simulink library "Source_Lib"  (R2017a)
settings: Solver=VariableStepAuto  StartTime=0.0  StopTime=10.0  RelTol=1e-3
undefined symbols (not defined in the file or in its folder): Cmu0, delta0, fb, GOV1_K2, ia0, ib0, Ib2, ic0, pha0, phb0, phc0, Theta0_deg, Time_Step, V0_pu, Vfu0
libraries: powerlib x41, Control_Lib x14, spsPower3phInstantaneousLib x3, spsSynchronousMachinepuFundamentalLib x2
(part 2 of 2)

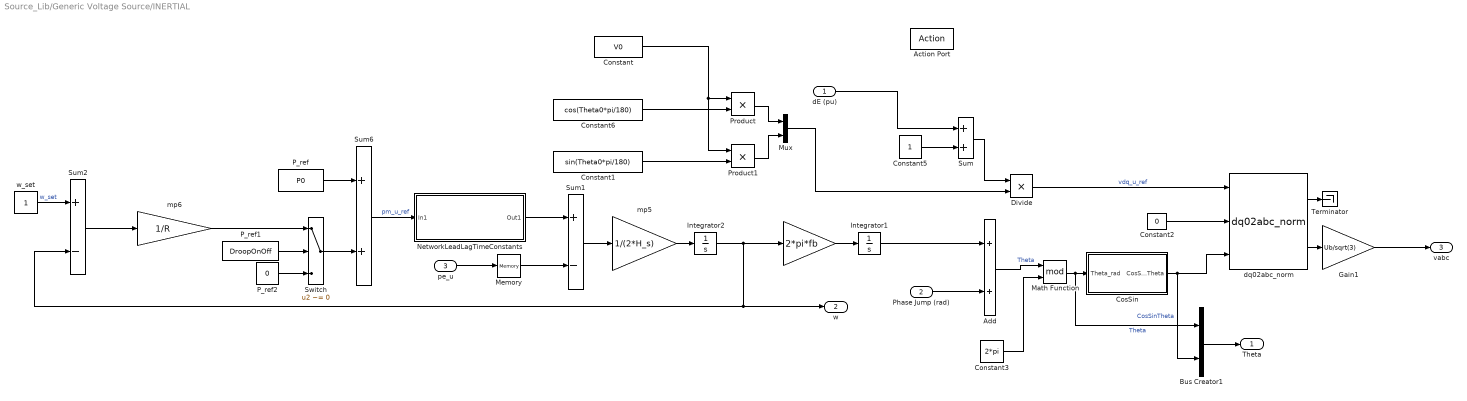
== system Source_Lib/Generic Voltage Source/INERTIAL ==
  dE (pu) : Inport
  Phase Jump (rad) : Inport  Port=2
  pe_u : Inport  Port=3
  Action Port : ActionPort
  " " : Gain  Gain=2*pi*fb
  Add : Sum
  Bus Creator1 : BusCreator  Inputs=2
  Constant : Constant  Value=V0
  Constant1 : Constant  Value=sin(Theta0*pi/180)
  Constant2 : Constant  Value=0
  Constant3 : Constant  Value=2*pi
  Constant5 : Constant
  Constant6 : Constant  Value=cos(Theta0*pi/180)
  CosSin : Subsystem
  Divide : Product  Inputs=**
  Gain1 : Gain  Gain=Ub/sqrt(3)
  Integrator1 : Integrator  InitialCondition=Theta0*pi/180
  Integrator2 : Integrator  InitialCondition=1
  Math Function : Math  Operator=mod  SaturateOnIntegerOverflow=on
  Memory : Memory
  Mux : Mux  Inputs=2
  NetworkLeadLagTimeConstants : Subsystem
  P_ref : Constant  Value=P0
  P_ref1 : Constant  Value=DroopOnOff
  P_ref2 : Constant  Value=0
  Product : Product
  Product1 : Product
  Sum : Sum
  Sum1 : Sum  Inputs=+-
  Sum2 : Sum  Inputs=+-
  Sum6 : Sum
  Switch : Switch  Criteria=u2 ~= 0
  Terminator : Terminator
  dq02abc_norm : Control_Lib/dq02abc_norm  referenceAxisMode=Reference axis at 90 degrees behind phase_a  baseUpdateGain=sqrt(3)
      settings: SourceProductName=VSC_Lib
  mp5 : Gain  Gain=1/(2*H_s)
  mp6 : Gain  Gain=1/R
  w_set : Constant
  Theta : Outport
  w : Outport  Port=2
  vabc : Outport  Port=3
  wires:
  dq02abc_norm/2 -> Gain1/1
  dE (pu)/1 -> Sum/1
  dq02abc_norm/1 -> Terminator/1
  Sum/1 -> Divide/1
  Gain1/1 -> vabc/1
  Product/1 -> Mux/1
  Constant6/1 -> Product/2
  Constant3/1 -> Math Function/2
  CosSin/1(CosSinTheta) -> Bus Creator1/2, dq02abc_norm/3  "CosSinTheta"
  Constant1/1 -> Product1/2
  Divide/1 -> dq02abc_norm/1  "vdq_u_ref"
  Constant/1 -> Product/1, Product1/1
  Phase Jump (rad)/1 -> Add/2
  Add/1 -> Math Function/1  "Theta"
  Math Function/1 -> Bus Creator1/1, CosSin/1(Theta_rad)  "Theta"
  Constant2/1 -> dq02abc_norm/2
  Product1/1 -> Mux/2
  Constant5/1 -> Sum/2
  Mux/1 -> Divide/2
  Bus Creator1/1 -> Theta/1
  NetworkLeadLagTimeConstants/1(Out1) -> Sum1/1
  P_ref/1 -> Sum6/1
  mp6/1 -> Switch/1
  " "/1 -> Integrator1/1
  Sum2/1 -> mp6/1
  P_ref2/1 -> Switch/3
  Integrator2/1 -> " "/1, Sum2/2, w/1
  P_ref1/1 -> Switch/2
  mp5/1 -> Integrator2/1
  pe_u/1 -> Memory/1
  Sum1/1 -> mp5/1
  Sum6/1 -> NetworkLeadLagTimeConstants/1(In1)  "pm_u_ref"
  Integrator1/1 -> Add/1
  Switch/1 -> Sum6/2
  w_set/1 -> Sum2/1  "w_set"
  Memory/1 -> Sum1/2

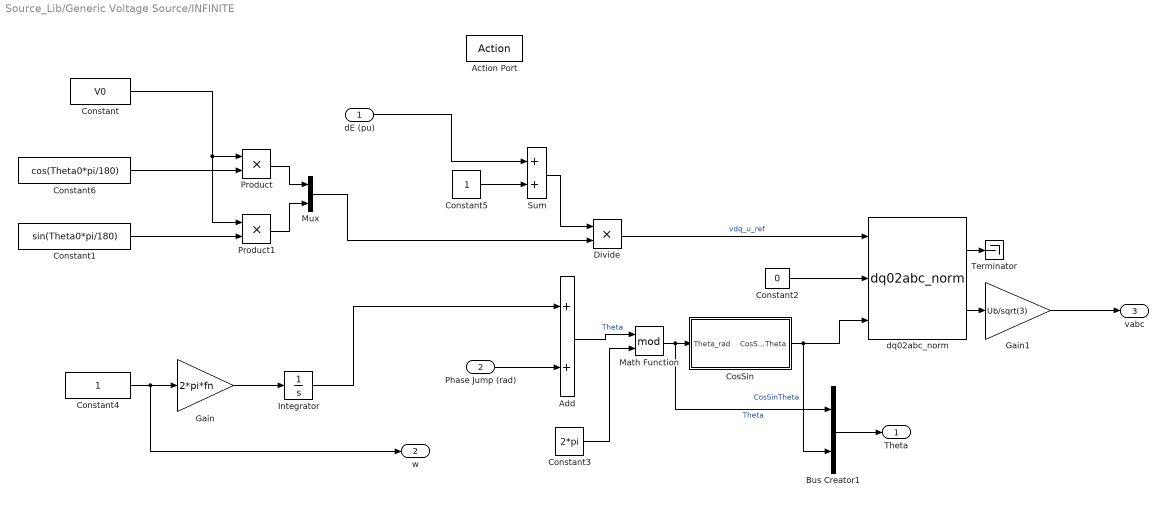
== system Source_Lib/Generic Voltage Source/INFINITE ==
  dE (pu) : Inport
  Phase Jump (rad) : Inport  Port=2
  Action Port : ActionPort
  Add : Sum
  Bus Creator1 : BusCreator  Inputs=2
  Constant : Constant  Value=V0
  Constant1 : Constant  Value=sin(Theta0*pi/180)
  Constant2 : Constant  Value=0
  Constant3 : Constant  Value=2*pi
  Constant4 : Constant
  Constant5 : Constant
  Constant6 : Constant  Value=cos(Theta0*pi/180)
  CosSin : Subsystem
  Divide : Product  Inputs=**
  Gain : Gain  Gain=2*pi*fn
  Gain1 : Gain  Gain=Ub/sqrt(3)
  Integrator : Integrator  InitialCondition=Theta0*pi/180
  Math Function : Math  Operator=mod  SaturateOnIntegerOverflow=on
  Mux : Mux  Inputs=2
  Product : Product
  Product1 : Product
  Sum : Sum
  Terminator : Terminator
  dq02abc_norm : Control_Lib/dq02abc_norm  referenceAxisMode=Reference axis at 90 degrees behind phase_a  baseUpdateGain=sqrt(3)
      settings: SourceProductName=VSC_Lib
  Theta : Outport
  w : Outport  Port=2
  vabc : Outport  Port=3
  wires:
  dq02abc_norm/2 -> Gain1/1
  Integrator/1 -> Add/1
  Gain/1 -> Integrator/1
  dE (pu)/1 -> Sum/1
  dq02abc_norm/1 -> Terminator/1
  Sum/1 -> Divide/1
  Constant4/1 -> w/1, Gain/1
  Gain1/1 -> vabc/1
  Product/1 -> Mux/1
  Constant6/1 -> Product/2
  Constant3/1 -> Math Function/2
  CosSin/1(CosSinTheta) -> Bus Creator1/2, dq02abc_norm/3  "CosSinTheta"
  Constant1/1 -> Product1/2
  Divide/1 -> dq02abc_norm/1  "vdq_u_ref"
  Constant/1 -> Product/1, Product1/1
  Phase Jump (rad)/1 -> Add/2
  Add/1 -> Math Function/1  "Theta"
  Math Function/1 -> Bus Creator1/1, CosSin/1(Theta_rad)  "Theta"
  Constant2/1 -> dq02abc_norm/2
  Product1/1 -> Mux/2
  Constant5/1 -> Sum/2
  Mux/1 -> Divide/2
  Bus Creator1/1 -> Theta/1

== system Source_Lib/Generic Voltage Source/Source_For_OP ==
  v_abc_ref : Inport
  Controlled Voltage Source1 : powerlib/Electrical Sources/Controlled Voltage Source  Initialize=off  Source_Type=AC  Amplitude=V0*Ub*sqrt(2/3)*sin(Theta0)  Phase=(Theta0*180/pi)  Frequency=fb  Measurements=None
  Controlled Voltage Source2 : powerlib/Electrical Sources/Controlled Voltage Source  Initialize=off  Source_Type=AC  Amplitude=V0*Ub*sqrt(2/3)*sin(Theta0-2*pi/3)  Phase=(Theta0*180/pi)-120  Frequency=fb  Measurements=None
  Controlled Voltage Source3 : powerlib/Electrical Sources/Controlled Voltage Source  Initialize=off  Source_Type=AC  Amplitude=V0*Ub*sqrt(2/3)*sin(Theta0-4*pi/3)  Phase=(Theta0*180/pi)+120  Frequency=fb  Measurements=None
  Demux : Demux  Outputs=3
  Step : Step  Time=1e-9  SampleTime=0
  Subsystem3 : Subsystem
  Three-Phase Source1 : powerlib/Electrical Sources/Three-Phase Source  InternalConnection=Yn  VoltagePhases=off  Voltage=V0*Ub  PhaseAngle=Theta0  Voltage_phases=[25e3 25e3 25e3]/sqrt(3)  PhaseAngles_phases=[0 -120 +120]  Frequency=fb  NonIdealSource=off  SpecifyImpedance=off  Resistance=0.8929  Inductance=16.58e-3  ShortCircuitLevel=100e6  BaseVoltage=25e3  XRratio=7  BusType=swing  Pref=10e3  Qref=0  Prefabc=[10e3, 10e3, 10e3]  Qrefabc=[0, 0, 0]  Qmin=-inf  Qmax=inf
  A : PMIOPort  Side=Right
  B : PMIOPort  Port=2  Side=Right
  C : PMIOPort  Port=3  Side=Right
  N : PMIOPort  Port=4  Side=Left
  wires:
  Step/1 -> Subsystem3/1(switch)
  Demux/3 -> Controlled Voltage Source3/1
  Demux/1 -> Controlled Voltage Source1/1
  v_abc_ref/1 -> Demux/1
  Demux/2 -> Controlled Voltage Source2/1
  connections:
  Three-Phase Source1/RConn3 -- Subsystem3/LConn6
  Three-Phase Source1/RConn2 -- Subsystem3/LConn5
  Three-Phase Source1/RConn1 -- Subsystem3/LConn4
  Controlled Voltage Source3/RConn1 -- Subsystem3/LConn3
  Controlled Voltage Source2/RConn1 -- Subsystem3/LConn2
  Controlled Voltage Source1/RConn1 -- Subsystem3/LConn1
  Subsystem3/RConn3 -- C/RConn1
  Subsystem3/RConn2 -- B/RConn1
  Subsystem3/RConn1 -- A/RConn1
  Controlled Voltage Source1/LConn1 -- Controlled Voltage Source2/LConn1 -- N/RConn1 -- Three-Phase Source1/LConn1 -- Controlled Voltage Source3/LConn1

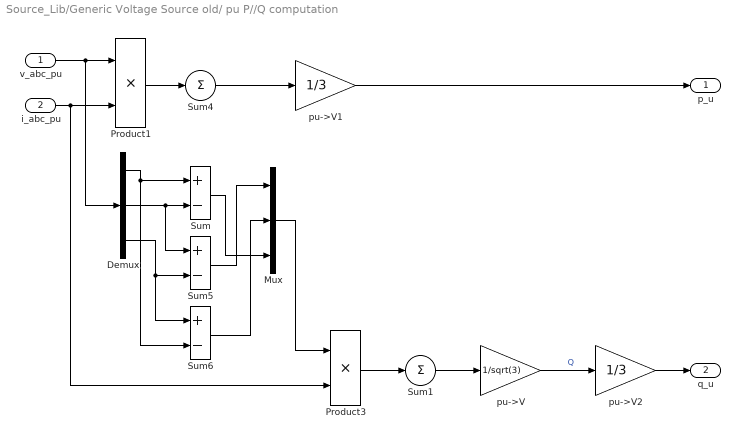
== system Source_Lib/Generic Voltage Source old/ pu P//Q computation ==
  v_abc_pu : Inport  PortDimensions=3
  i_abc_pu : Inport  Port=2  PortDimensions=3
  Demux : Demux  Outputs=3
      settings: DisplayOption=none
  Mux : Mux  Inputs=3
  Product1 : Product  InputSameDT=on  SaturateOnIntegerOverflow=on  OutDataTypeStr=Inherit: Same as first input
  Product3 : Product  InputSameDT=on  SaturateOnIntegerOverflow=on  OutDataTypeStr=Inherit: Same as first input
  Sum : Sum  Inputs=+-  InputSameDT=on  SaturateOnIntegerOverflow=on  OutDataTypeStr=Inherit: Same as first input
  Sum1 : Sum  Inputs=1  InputSameDT=on  SaturateOnIntegerOverflow=on  OutDataTypeStr=Inherit: Same as first input
  Sum4 : Sum  Inputs=1  InputSameDT=on  SaturateOnIntegerOverflow=on  OutDataTypeStr=Inherit: Same as first input
  Sum5 : Sum  Inputs=+-  InputSameDT=on  SaturateOnIntegerOverflow=on  OutDataTypeStr=Inherit: Same as first input
  Sum6 : Sum  Inputs=+-  InputSameDT=on  SaturateOnIntegerOverflow=on  OutDataTypeStr=Inherit: Same as first input
  pu->V : Gain  Gain=1/sqrt(3)  SaturateOnIntegerOverflow=on  OutDataTypeStr=Inherit: Same as input  ParamDataTypeStr=Inherit: Same as input
  pu->V1 : Gain  Gain=1/3  SaturateOnIntegerOverflow=on  OutDataTypeStr=Inherit: Same as input  ParamDataTypeStr=Inherit: Same as input
  pu->V2 : Gain  Gain=1/3  SaturateOnIntegerOverflow=on  OutDataTypeStr=Inherit: Same as input  ParamDataTypeStr=Inherit: Same as input
  p_u : Outport
  q_u : Outport  Port=2
  wires:
  pu->V2/1 -> q_u/1
  pu->V1/1 -> p_u/1
  Sum1/1 -> pu->V/1
  Product3/1 -> Sum1/1
  Product1/1 -> Sum4/1
  v_abc_pu/1 -> Product1/1, Demux/1
  i_abc_pu/1 -> Product1/2, Product3/2
  Sum4/1 -> pu->V1/1
  Demux/1 -> Sum/1, Sum6/2
  Demux/2 -> Sum/2, Sum5/1
  Demux/3 -> Sum5/2, Sum6/1
  Sum/1 -> Mux/3
  Sum5/1 -> Mux/1
  Sum6/1 -> Mux/2
  Mux/1 -> Product3/1
  pu->V/1 -> pu->V2/1  "Q"

== system Source_Lib/Generic Voltage Source old/CosSin ==
  Theta_rad : Inport
  Mux : Mux  Inputs=2
  Trigonometric Function : Trigonometry
  Trigonometric Function1 : Trigonometry  Operator=cos
  CosSinTheta : Outport
  wires:
  Theta_rad/1 -> Trigonometric Function/1, Trigonometric Function1/1
  Trigonometric Function/1 -> Mux/2
  Mux/1 -> CosSinTheta/1
  Trigonometric Function1/1 -> Mux/1

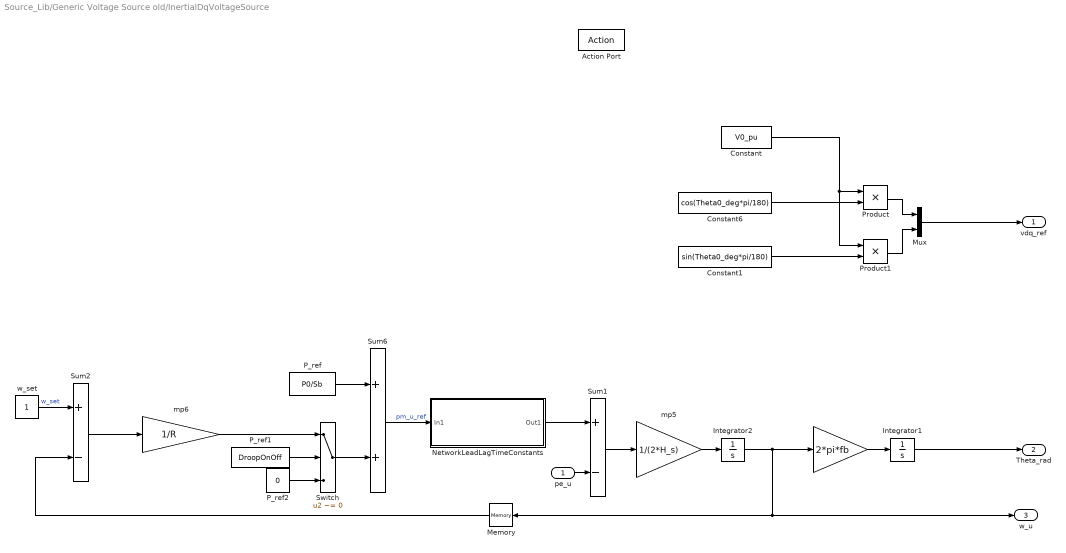
== system Source_Lib/Generic Voltage Source old/InertialDqVoltageSource ==
  pe_u : Inport
  Action Port : ActionPort
  " " : Gain  Gain=2*pi*fb
  Constant : Constant  Value=V0_pu
  Constant1 : Constant  Value=sin(Theta0_deg*pi/180)
  Constant6 : Constant  Value=cos(Theta0_deg*pi/180)
  Integrator1 : Integrator  InitialCondition=Theta0_deg*pi/180
  Integrator2 : Integrator  InitialCondition=1
  Memory : Memory  X0=1
  Mux : Mux  Inputs=2
  NetworkLeadLagTimeConstants : Subsystem
  P_ref : Constant  Value=P0/Sb
  P_ref1 : Constant  Value=DroopOnOff
  P_ref2 : Constant  Value=0
  Product : Product
  Product1 : Product
  Sum1 : Sum  Inputs=+-
  Sum2 : Sum  Inputs=+-
  Sum6 : Sum
  Switch : Switch  Criteria=u2 ~= 0
  mp5 : Gain  Gain=1/(2*H_s)
  mp6 : Gain  Gain=1/R
  w_set : Constant
  vdq_ref : Outport
  Theta_rad : Outport  Port=2
  w_u : Outport  Port=3
  wires:
  mp5/1 -> Integrator2/1
  Sum6/1 -> NetworkLeadLagTimeConstants/1(In1)  "pm_u_ref"
  Integrator2/1 -> w_u/1, Memory/1, " "/1
  P_ref/1 -> Sum6/1
  Sum2/1 -> mp6/1
  Sum1/1 -> mp5/1
  " "/1 -> Integrator1/1
  pe_u/1 -> Sum1/2
  w_set/1 -> Sum2/1  "w_set"
  Integrator1/1 -> Theta_rad/1
  Constant1/1 -> Product1/2
  Constant6/1 -> Product/2
  Constant/1 -> Product1/1, Product/1
  Product1/1 -> Mux/2
  Product/1 -> Mux/1
  Mux/1 -> vdq_ref/1
  NetworkLeadLagTimeConstants/1(Out1) -> Sum1/1
  P_ref1/1 -> Switch/2
  Switch/1 -> Sum6/2
  mp6/1 -> Switch/1
  P_ref2/1 -> Switch/3
  Memory/1 -> Sum2/2

== system Source_Lib/Generic Voltage Source old/InfiniteDqVoltageSource ==
  Action Port : ActionPort
  Constant : Constant  Value=V0_pu
  Constant1 : Constant  Value=sin(Theta0_deg*pi/180)
  Constant4 : Constant
  Constant6 : Constant  Value=cos(Theta0_deg*pi/180)
  Gain : Gain  Gain=2*pi*fn
  Integrator : Integrator  InitialCondition=Theta0_deg*pi/180
  Mux : Mux  Inputs=2
  Product : Product
  Product1 : Product
  vdq_u_ref : Outport
  Theta_rad : Outport  Port=2
  w_u : Outport  Port=3
  wires:
  Constant1/1 -> Product1/2
  Gain/1 -> Integrator/1
  Product/1 -> Mux/1
  Constant6/1 -> Product/2
  Constant/1 -> Product1/1, Product/1
  Product1/1 -> Mux/2
  Integrator/1 -> Theta_rad/1
  Mux/1 -> vdq_u_ref/1
  Constant4/1 -> w_u/1, Gain/1

== system Source_Lib/Generic Voltage Source old/Source_For_OP ==
  v_abc_ref : Inport
  Controlled Voltage Source1 : powerlib/Electrical Sources/Controlled Voltage Source  Initialize=off  Source_Type=AC  Amplitude=V0*Ub*sqrt(2/3)*sin(Theta0)  Phase=(Theta0*180/pi)  Frequency=fb  Measurements=None
  Controlled Voltage Source2 : powerlib/Electrical Sources/Controlled Voltage Source  Initialize=off  Source_Type=AC  Amplitude=V0*Ub*sqrt(2/3)*sin(Theta0-2*pi/3)  Phase=(Theta0*180/pi)-120  Frequency=fb  Measurements=None
  Controlled Voltage Source3 : powerlib/Electrical Sources/Controlled Voltage Source  Initialize=off  Source_Type=AC  Amplitude=V0*Ub*sqrt(2/3)*sin(Theta0-4*pi/3)  Phase=(Theta0*180/pi)+120  Frequency=fb  Measurements=None
  Demux : Demux  Outputs=3
  Step : Step  Time=1e-9  SampleTime=0
  Subsystem3 : Subsystem
  Three-Phase Source1 : powerlib/Electrical Sources/Three-Phase Source  InternalConnection=Yn  VoltagePhases=off  Voltage=V0_pu*Ub  PhaseAngle=Theta0_deg  Voltage_phases=[25e3 25e3 25e3]/sqrt(3)  PhaseAngles_phases=[0 -120 +120]  Frequency=fb  NonIdealSource=off  SpecifyImpedance=off  Resistance=0.8929  Inductance=16.58e-3  ShortCircuitLevel=100e6  BaseVoltage=25e3  XRratio=7  BusType=swing  Pref=10e3  Qref=0  Prefabc=[10e3, 10e3, 10e3]  Qrefabc=[0, 0, 0]  Qmin=-inf  Qmax=inf
  A : PMIOPort  Side=Right
  B : PMIOPort  Port=2  Side=Right
  C : PMIOPort  Port=3  Side=Right
  N : PMIOPort  Port=4  Side=Left
  wires:
  Demux/2 -> Controlled Voltage Source2/1
  v_abc_ref/1 -> Demux/1
  Demux/1 -> Controlled Voltage Source1/1
  Demux/3 -> Controlled Voltage Source3/1
  Step/1 -> Subsystem3/1(switch)
  connections:
  Controlled Voltage Source3/LConn1 -- Three-Phase Source1/LConn1 -- N/RConn1 -- Controlled Voltage Source2/LConn1 -- Controlled Voltage Source1/LConn1
  Subsystem3/RConn1 -- A/RConn1
  Subsystem3/RConn2 -- B/RConn1
  Subsystem3/RConn3 -- C/RConn1
  Controlled Voltage Source1/RConn1 -- Subsystem3/LConn1
  Controlled Voltage Source2/RConn1 -- Subsystem3/LConn2
  Controlled Voltage Source3/RConn1 -- Subsystem3/LConn3
  Three-Phase Source1/RConn1 -- Subsystem3/LConn4
  Three-Phase Source1/RConn2 -- Subsystem3/LConn5
  Three-Phase Source1/RConn3 -- Subsystem3/LConn6

== system Source_Lib/Synchronous Machine with control and transformer/EX ==
  OP_Vfu : Inport
  Vtdq : Inport  Port=2
  Vref : Inport  Port=3
  vstab : Inport  Port=4
  Filter : Subsystem  mask{K=1, tau=ST1_taur, init_value=V0}
      mask prompts: K "Gain"; tau "Time Constant"; init_value "Initial Value"
  Gain : Gain  Gain=ST1_Ka
  Gain1 : Gain  Gain=1/ST1_Ka
  Module1 : Subsystem
  Sum : Sum  Inputs=+-+-
  Vfu : Outport
  wires:
  Gain/1 -> Vfu/1
  vstab/1 -> Sum/4
  Vtdq/1 -> Module1/1(x)
  Gain1/1 -> Sum/1
  Sum/1 -> Gain/1
  OP_Vfu/1 -> Gain1/1
  Vref/1 -> Sum/3
  Filter/1(Output) -> Sum/2
  Module1/1(||x||) -> Filter/1(In1)

== system Source_Lib/Synchronous Machine with control and transformer/Governor + Turbine ==
  Pref : Inport
  wr : Inport  Port=2
  wg : Inport  Port=3
  Gain : Gain  Gain=1-GOV_K3
  Gain1 : Gain  Gain=1-GOV_K2
  GovernorP1 : TransferFcn  Numerator=[GOV_Kpf]  Denominator=[GOV_tau1 1]
  GovernorP2 : TransferFcn  Denominator=[GOV_tau3 1]
  Reheater IP : Subsystem  mask{K=GOV_K2, tau=GOV_tau5, init_value=Cmu0*GOV_K2}
      mask prompts: K "Gain"; tau "Time Constant"; init_value "Initial Value"
  Reheater LP : Subsystem  mask{K=GOV_K3, tau=GOV_tau6, init_value=Cmu0*GOV_K2*GOV_K3}
      mask prompts: K "Gain"; tau "Time Constant"; init_value "Initial Value"
  Saturation : Saturate  UpperLimit=1  LowerLimit=0
  Sum : Sum  Inputs=-+|
  Sum1 : Sum  Inputs=+-|
  Sum2 : Sum  Inputs=+++
  Valve : Subsystem  mask{K=1, tau=GOV_tau4, init_value=Cmu0}
      mask prompts: K "Gain"; tau "Time Constant"; init_value "Initial Value"
      mask Display: disp('valve')
  cmu in : Outport
  wires:
  Pref/1 -> Sum1/1
  Saturation/1 -> Valve/1(Pm*)
  wr/1 -> Sum/1
  Sum1/1 -> Saturation/1
  Reheater LP/1(Output) -> Sum2/3  "P_lp"
  Gain1/1 -> Sum2/1  "P_hp"
  Gain/1 -> Sum2/2  "P_ip"
  Reheater IP/1(Output) -> Reheater LP/1(In1), Gain/1
  Valve/1(Pm) -> Reheater IP/1(In1), Gain1/1
  Sum2/1 -> cmu in/1
  Sum/1 -> GovernorP1/1
  GovernorP2/1 -> Sum1/2
  GovernorP1/1 -> GovernorP2/1
  wg/1 -> Sum/2

== system Source_Lib/Synchronous Machine with control and transformer/PSS ==
  wr : Inport
  Add1 : Sum  Inputs=-+|
  Constant : Constant
  Gain : Gain  Gain=PSS_K
  P : TransferFcn  Denominator=[PSS_tau6 1]
  Phase compensator 1 : TransferFcn  Numerator=[PSS_tau1 1]  Denominator=[PSS_tau2 1]
  Phase compensator 2 : TransferFcn  Numerator=[PSS_tau3 1]  Denominator=[PSS_tau4 1]
  "Washout\t" : TransferFcn  Numerator=[PSS_tau5 0]  Denominator=[PSS_tau5 1]
  vstab : Outport
  wires:
  Constant/1 -> Add1/2
  P/1 -> Gain/1
  wr/1 -> Add1/1
  Phase compensator 1/1 -> Phase compensator 2/1
  Gain/1 -> "Washout\t"/1
  Phase compensator 2/1 -> vstab/1
  Add1/1 -> P/1
  "Washout\t"/1 -> Phase compensator 1/1

== system Source_Lib/Synchronous Machine with control and transformer old/EX ==
  OP_Vfu : Inport
  Vtdq : Inport  Port=2
  Vref : Inport  Port=3
  vstab : Inport  Port=4
  Filter : Subsystem  mask{K=1, tau=ST1_taur, init_value=V0}
      mask prompts: K "Gain"; tau "Time Constant"; init_value "Initial Value"
  Gain : Gain  Gain=ST1_Ka
  Gain1 : Gain  Gain=1/ST1_Ka
  Module1 : Subsystem
  Sum : Sum  Inputs=+-+-
  Vfu : Outport
  wires:
  Module1/1(||x||) -> Filter/1(In1)
  Filter/1(Output) -> Sum/2
  Vref/1 -> Sum/3
  OP_Vfu/1 -> Gain1/1
  Sum/1 -> Gain/1
  Gain1/1 -> Sum/1
  Vtdq/1 -> Module1/1(x)
  vstab/1 -> Sum/4
  Gain/1 -> Vfu/1

== system Source_Lib/Synchronous Machine with control and transformer old/Governor + Turbine ==
  Pref : Inport
  wr : Inport  Port=2
  wg : Inport  Port=3
  Gain : Gain  Gain=1-GOV_K3
  Gain1 : Gain  Gain=1-GOV1_K2
  GovernorP1 : TransferFcn  Numerator=[GOV_Kpf]  Denominator=[GOV_tau1 1]
  GovernorP2 : TransferFcn  Denominator=[GOV_tau3 1]
  Reheater IP : Subsystem  mask{K=GOV_K2, tau=GOV_tau5, init_value=Cmu0*GOV_K2}
      mask prompts: K "Gain"; tau "Time Constant"; init_value "Initial Value"
  Reheater LP : Subsystem  mask{K=GOV_K3, tau=GOV_tau6, init_value=Cmu0*GOV_K2*GOV_K3}
      mask prompts: K "Gain"; tau "Time Constant"; init_value "Initial Value"
  Saturation : Saturate  UpperLimit=1  LowerLimit=0
  Sum : Sum  Inputs=-+|
  Sum1 : Sum  Inputs=+-|
  Sum2 : Sum  Inputs=+++
  Valve : Subsystem  mask{K=1, tau=GOV_tau4, init_value=Cmu0}
      mask prompts: K "Gain"; tau "Time Constant"; init_value "Initial Value"
      mask Display: disp('valve')
  cmu in : Outport
  wires:
  wg/1 -> Sum/2
  GovernorP1/1 -> GovernorP2/1
  GovernorP2/1 -> Sum1/2
  Sum/1 -> GovernorP1/1
  Sum2/1 -> cmu in/1
  Valve/1(Pm) -> Gain1/1, Reheater IP/1(In1)
  Reheater IP/1(Output) -> Gain/1, Reheater LP/1(In1)
  Gain/1 -> Sum2/2  "P_ip"
  Gain1/1 -> Sum2/1  "P_hp"
  Reheater LP/1(Output) -> Sum2/3  "P_lp"
  Sum1/1 -> Saturation/1
  wr/1 -> Sum/1
  Saturation/1 -> Valve/1(Pm*)
  Pref/1 -> Sum1/1

== system Source_Lib/Synchronous Machine with control and transformer old/PSS ==
  wr : Inport
  Add1 : Sum  Inputs=-+|
  Constant : Constant
  Gain : Gain  Gain=PSS_K
  P : TransferFcn  Denominator=[PSS_tau6 1]
  Phase compensator 1 : TransferFcn  Numerator=[PSS_tau1 1]  Denominator=[PSS_tau2 1]
  Phase compensator 2 : TransferFcn  Numerator=[PSS_tau3 1]  Denominator=[PSS_tau4 1]
  "Washout\t" : TransferFcn  Numerator=[PSS_tau5 0]  Denominator=[PSS_tau5 1]
  vstab : Outport
  wires:
  "Washout\t"/1 -> Phase compensator 1/1
  Add1/1 -> P/1
  Phase compensator 2/1 -> vstab/1
  Gain/1 -> "Washout\t"/1
  Phase compensator 1/1 -> Phase compensator 2/1
  wr/1 -> Add1/1
  P/1 -> Gain/1
  Constant/1 -> Add1/2

== system Source_Lib/Generic Voltage Source/INERTIAL/CosSin ==
  Theta_rad : Inport
  Mux : Mux  Inputs=2
  Trigonometric Function : Trigonometry
  Trigonometric Function1 : Trigonometry  Operator=cos
  CosSinTheta : Outport
  wires:
  Theta_rad/1 -> Trigonometric Function/1, Trigonometric Function1/1
  Trigonometric Function/1 -> Mux/2
  Mux/1 -> CosSinTheta/1
  Trigonometric Function1/1 -> Mux/1

== system Source_Lib/Generic Voltage Source/INERTIAL/NetworkLeadLagTimeConstants ==
  In1 : Inport
  Constant : Constant  Value=P0
  Integrator3 : Integrator  InitialConditionSource=external  InitialCondition=(P0/Sb)*(1-TN/TD)
  Sum1 : Sum
  Sum2 : Sum  Inputs=+-
  Sum3 : Sum  Inputs=-+
  mp1 : Gain  Gain=TN/TD
  mp2 : Gain  Gain=1-TN/TD
  mp3 : Gain  Gain=1/TD
  Out1 : Outport
  wires:
  Sum1/1 -> Out1/1
  mp1/1 -> Sum3/1, Sum1/1
  mp2/1 -> Sum2/1
  In1/1 -> mp2/1, mp1/1
  mp3/1 -> Integrator3/1
  Sum2/1 -> mp3/1
  Constant/1 -> Sum3/2
  Integrator3/1 -> Sum1/2, Sum2/2
  Sum3/1 -> Integrator3/2

== system Source_Lib/Generic Voltage Source/INFINITE/CosSin ==
  Theta_rad : Inport
  Mux : Mux  Inputs=2
  Trigonometric Function : Trigonometry
  Trigonometric Function1 : Trigonometry  Operator=cos
  CosSinTheta : Outport
  wires:
  Theta_rad/1 -> Trigonometric Function/1, Trigonometric Function1/1
  Trigonometric Function/1 -> Mux/2
  Mux/1 -> CosSinTheta/1
  Trigonometric Function1/1 -> Mux/1

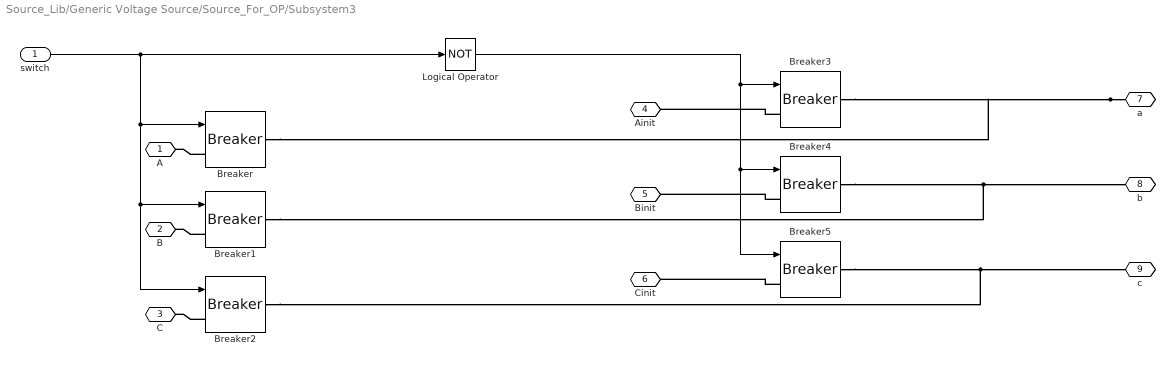
== system Source_Lib/Generic Voltage Source/Source_For_OP/Subsystem3 ==
  switch : Inport
  Breaker : powerlib/Elements/Breaker  InitialState=0  SwitchingTimes="[1/60  5/60]"  External=on  BreakerResistance=0.001  SnubberResistance=1e6  SnubberCapacitance=inf  Measurements=None  MoreParameters=on  NoBreakLoop=off
  Breaker1 : powerlib/Elements/Breaker  InitialState=0  SwitchingTimes="[1/60  5/60]"  External=on  BreakerResistance=0.001  SnubberResistance=1e6  SnubberCapacitance=inf  Measurements=None  MoreParameters=on  NoBreakLoop=off
  Breaker2 : powerlib/Elements/Breaker  InitialState=0  SwitchingTimes="[1/60  5/60]"  External=on  BreakerResistance=0.001  SnubberResistance=1e6  SnubberCapacitance=inf  Measurements=None  MoreParameters=on  NoBreakLoop=off
  Breaker3 : powerlib/Elements/Breaker  InitialState=1  SwitchingTimes="[1/60  5/60]"  External=on  BreakerResistance=0.001  SnubberResistance=1e6  SnubberCapacitance=inf  Measurements=None  MoreParameters=on  NoBreakLoop=off
  Breaker4 : powerlib/Elements/Breaker  InitialState=1  SwitchingTimes="[1/60  5/60]"  External=on  BreakerResistance=0.001  SnubberResistance=1e6  SnubberCapacitance=inf  Measurements=None  MoreParameters=on  NoBreakLoop=off
  Breaker5 : powerlib/Elements/Breaker  InitialState=1  SwitchingTimes="[1/60  5/60]"  External=on  BreakerResistance=0.001  SnubberResistance=1e6  SnubberCapacitance=inf  Measurements=None  MoreParameters=on  NoBreakLoop=off
  Logical Operator : Logic  Operator=NOT  AllPortsSameDT=off  OutDataTypeStr=boolean
  A : PMIOPort  Side=Left
  B : PMIOPort  Port=2  Side=Left
  C : PMIOPort  Port=3  Side=Left
  Ainit : PMIOPort  Port=4  Side=Left
  Binit : PMIOPort  Port=5  Side=Left
  Cinit : PMIOPort  Port=6  Side=Left
  a : PMIOPort  Port=7  Side=Right
  b : PMIOPort  Port=8  Side=Right
  c : PMIOPort  Port=9  Side=Right
  wires:
  Logical Operator/1 -> Breaker3/1, Breaker4/1, Breaker5/1
  switch/1 -> Logical Operator/1, Breaker/1, Breaker1/1, Breaker2/1
  connections:
  Breaker4/RConn1 -- Breaker1/RConn1 -- b/RConn1
  a/RConn1 -- Breaker3/RConn1 -- Breaker/RConn1
  Breaker1/LConn1 -- B/RConn1
  Breaker3/LConn1 -- Ainit/RConn1
  Breaker2/LConn1 -- C/RConn1
  Breaker4/LConn1 -- Binit/RConn1
  Breaker2/RConn1 -- Breaker5/RConn1 -- c/RConn1
  Breaker5/LConn1 -- Cinit/RConn1
  Breaker/LConn1 -- A/RConn1

== system Source_Lib/Generic Voltage Source old/InertialDqVoltageSource/NetworkLeadLagTimeConstants ==
  In1 : Inport
  Integrator3 : Integrator  InitialCondition=(P0/Sb)*(1-TN/TD)
  Sum1 : Sum
  Sum2 : Sum  Inputs=+-
  mp1 : Gain  Gain=TN/TD
  mp2 : Gain  Gain=1-TN/TD
  mp3 : Gain  Gain=1/TD
  Out1 : Outport
  wires:
  Sum1/1 -> Out1/1
  mp1/1 -> Sum1/1
  mp2/1 -> Sum2/1
  In1/1 -> mp2/1, mp1/1
  Integrator3/1 -> Sum2/2, Sum1/2
  mp3/1 -> Integrator3/1
  Sum2/1 -> mp3/1

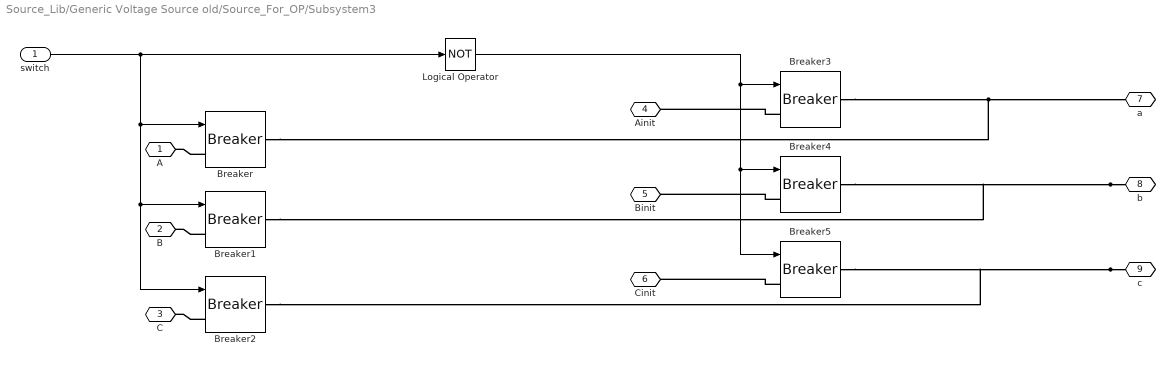
== system Source_Lib/Generic Voltage Source old/Source_For_OP/Subsystem3 ==
  switch : Inport
  Breaker : powerlib/Elements/Breaker  InitialState=0  SwitchingTimes="[1/60  5/60]"  External=on  BreakerResistance=0.001  SnubberResistance=1e6  SnubberCapacitance=inf  Measurements=None  MoreParameters=on  NoBreakLoop=off
  Breaker1 : powerlib/Elements/Breaker  InitialState=0  SwitchingTimes="[1/60  5/60]"  External=on  BreakerResistance=0.001  SnubberResistance=1e6  SnubberCapacitance=inf  Measurements=None  MoreParameters=on  NoBreakLoop=off
  Breaker2 : powerlib/Elements/Breaker  InitialState=0  SwitchingTimes="[1/60  5/60]"  External=on  BreakerResistance=0.001  SnubberResistance=1e6  SnubberCapacitance=inf  Measurements=None  MoreParameters=on  NoBreakLoop=off
  Breaker3 : powerlib/Elements/Breaker  InitialState=1  SwitchingTimes="[1/60  5/60]"  External=on  BreakerResistance=0.001  SnubberResistance=1e6  SnubberCapacitance=inf  Measurements=None  MoreParameters=on  NoBreakLoop=off
  Breaker4 : powerlib/Elements/Breaker  InitialState=1  SwitchingTimes="[1/60  5/60]"  External=on  BreakerResistance=0.001  SnubberResistance=1e6  SnubberCapacitance=inf  Measurements=None  MoreParameters=on  NoBreakLoop=off
  Breaker5 : powerlib/Elements/Breaker  InitialState=1  SwitchingTimes="[1/60  5/60]"  External=on  BreakerResistance=0.001  SnubberResistance=1e6  SnubberCapacitance=inf  Measurements=None  MoreParameters=on  NoBreakLoop=off
  Logical Operator : Logic  Operator=NOT  AllPortsSameDT=off  OutDataTypeStr=boolean
  A : PMIOPort  Side=Left
  B : PMIOPort  Port=2  Side=Left
  C : PMIOPort  Port=3  Side=Left
  Ainit : PMIOPort  Port=4  Side=Left
  Binit : PMIOPort  Port=5  Side=Left
  Cinit : PMIOPort  Port=6  Side=Left
  a : PMIOPort  Port=7  Side=Right
  b : PMIOPort  Port=8  Side=Right
  c : PMIOPort  Port=9  Side=Right
  wires:
  switch/1 -> Breaker2/1, Breaker1/1, Breaker/1, Logical Operator/1
  Logical Operator/1 -> Breaker5/1, Breaker4/1, Breaker3/1
  connections:
  Breaker/LConn1 -- A/RConn1
  Breaker5/LConn1 -- Cinit/RConn1
  c/RConn1 -- Breaker5/RConn1 -- Breaker2/RConn1
  Breaker4/LConn1 -- Binit/RConn1
  Breaker2/LConn1 -- C/RConn1
  Breaker3/LConn1 -- Ainit/RConn1
  Breaker1/LConn1 -- B/RConn1
  Breaker/RConn1 -- Breaker3/RConn1 -- a/RConn1
  b/RConn1 -- Breaker1/RConn1 -- Breaker4/RConn1

== system Source_Lib/Synchronous Machine with control and transformer/EX/Filter ==
  In1 : Inport
  Gain : Gain  Gain=K
  Gain3 : Gain  Gain=1/tau
  Integrator : Integrator  InitialCondition=init_value/K
  Sum3 : Sum  Inputs=|+-
  Output : Outport
  wires:
  Gain3/1 -> Integrator/1
  Gain/1 -> Output/1
  Integrator/1 -> Gain/1, Sum3/2
  Sum3/1 -> Gain3/1
  In1/1 -> Sum3/1

== system Source_Lib/Synchronous Machine with control and transformer/EX/Module1 ==
  x : Inport
  Add1 : Sum
  Demux : Demux  Outputs=2
  Math Function : Math  Operator=square  SaturateOnIntegerOverflow=on
  Math Function1 : Math  Operator=square  SaturateOnIntegerOverflow=on
  Sqrt : Sqrt  SaturateOnIntegerOverflow=on
  ||x|| : Outport
  wires:
  Demux/1 -> Math Function/1
  Add1/1 -> Sqrt/1
  Math Function/1 -> Add1/1
  Math Function1/1 -> Add1/2
  x/1 -> Demux/1
  Sqrt/1 -> ||x||/1
  Demux/2 -> Math Function1/1

== system Source_Lib/Synchronous Machine with control and transformer/Governor + Turbine/Reheater IP ==
  In1 : Inport
  Constant : Constant  Value=init_value/K
  Gain : Gain  Gain=K
  Gain3 : Gain  Gain=1/tau
  Integrator : Integrator  InitialConditionSource=external
  Sum3 : Sum  Inputs=|+-
  Output : Outport
  wires:
  Gain3/1 -> Integrator/1
  Gain/1 -> Output/1
  Integrator/1 -> Gain/1, Sum3/2
  Sum3/1 -> Gain3/1
  In1/1 -> Sum3/1
  Constant/1 -> Integrator/2

== system Source_Lib/Synchronous Machine with control and transformer/Governor + Turbine/Reheater LP ==
  In1 : Inport
  Constant : Constant  Value=init_value/K
  Gain : Gain  Gain=K
  Gain3 : Gain  Gain=1/tau
  Integrator : Integrator  InitialConditionSource=external
  Sum3 : Sum  Inputs=|+-
  Output : Outport
  wires:
  In1/1 -> Sum3/1
  Sum3/1 -> Gain3/1
  Integrator/1 -> Gain/1, Sum3/2
  Gain/1 -> Output/1
  Gain3/1 -> Integrator/1
  Constant/1 -> Integrator/2

== system Source_Lib/Synchronous Machine with control and transformer/Governor + Turbine/Valve ==
  Pm* : Inport
  Constant : Constant  Value=init_value/K
  Gain : Gain  Gain=K
  Gain3 : Gain  Gain=1/tau
  Integrator : Integrator  InitialConditionSource=external
  Sum3 : Sum  Inputs=|+-
  Pm : Outport
  wires:
  Pm*/1 -> Sum3/1
  Sum3/1 -> Gain3/1
  Integrator/1 -> Gain/1, Sum3/2
  Gain/1 -> Pm/1
  Gain3/1 -> Integrator/1
  Constant/1 -> Integrator/2

== system Source_Lib/Synchronous Machine with control and transformer old/EX/Filter ==
  In1 : Inport
  Gain : Gain  Gain=K
  Gain3 : Gain  Gain=1/tau
  Integrator : Integrator  InitialCondition=init_value/K
  Sum3 : Sum  Inputs=|+-
  Output : Outport
  wires:
  In1/1 -> Sum3/1
  Sum3/1 -> Gain3/1
  Integrator/1 -> Sum3/2, Gain/1
  Gain/1 -> Output/1
  Gain3/1 -> Integrator/1

== system Source_Lib/Synchronous Machine with control and transformer old/EX/Module1 ==
  x : Inport
  Add1 : Sum
  Demux : Demux  Outputs=2
  Math Function : Math  Operator=square  SaturateOnIntegerOverflow=on
  Math Function1 : Math  Operator=square  SaturateOnIntegerOverflow=on
  Sqrt : Sqrt  SaturateOnIntegerOverflow=on
  ||x|| : Outport
  wires:
  Demux/2 -> Math Function1/1
  Sqrt/1 -> ||x||/1
  x/1 -> Demux/1
  Math Function1/1 -> Add1/2
  Math Function/1 -> Add1/1
  Add1/1 -> Sqrt/1
  Demux/1 -> Math Function/1

== system Source_Lib/Synchronous Machine with control and transformer old/Governor + Turbine/Reheater IP ==
  In1 : Inport
  Constant : Constant  Value=init_value/K
  Gain : Gain  Gain=K
  Gain3 : Gain  Gain=1/tau
  Integrator : Integrator  InitialConditionSource=external
  Sum3 : Sum  Inputs=|+-
  Output : Outport
  wires:
  Constant/1 -> Integrator/2
  In1/1 -> Sum3/1
  Sum3/1 -> Gain3/1
  Integrator/1 -> Sum3/2, Gain/1
  Gain/1 -> Output/1
  Gain3/1 -> Integrator/1

== system Source_Lib/Synchronous Machine with control and transformer old/Governor + Turbine/Reheater LP ==
  In1 : Inport
  Constant : Constant  Value=init_value/K
  Gain : Gain  Gain=K
  Gain3 : Gain  Gain=1/tau
  Integrator : Integrator  InitialConditionSource=external
  Sum3 : Sum  Inputs=|+-
  Output : Outport
  wires:
  Constant/1 -> Integrator/2
  Gain3/1 -> Integrator/1
  Gain/1 -> Output/1
  Integrator/1 -> Sum3/2, Gain/1
  Sum3/1 -> Gain3/1
  In1/1 -> Sum3/1

== system Source_Lib/Synchronous Machine with control and transformer old/Governor + Turbine/Valve ==
  Pm* : Inport
  Constant : Constant  Value=init_value/K
  Gain : Gain  Gain=K
  Gain3 : Gain  Gain=1/tau
  Integrator : Integrator  InitialConditionSource=external
  Sum3 : Sum  Inputs=|+-
  Pm : Outport
  wires:
  Constant/1 -> Integrator/2
  Gain3/1 -> Integrator/1
  Gain/1 -> Pm/1
  Integrator/1 -> Sum3/2, Gain/1
  Sum3/1 -> Gain3/1
  Pm*/1 -> Sum3/1
